simulink model "Q2"  (R2020b)
settings: Solver=VariableStepAuto  StartTime=0.0  StopTime=30  RelTol=1e-3
undefined symbols (not defined in the file): A_num, B_num, C_num, K_fast, K_slow
libraries: simulink x2
settings Model: Creator=asus  LastModifiedBy=asus

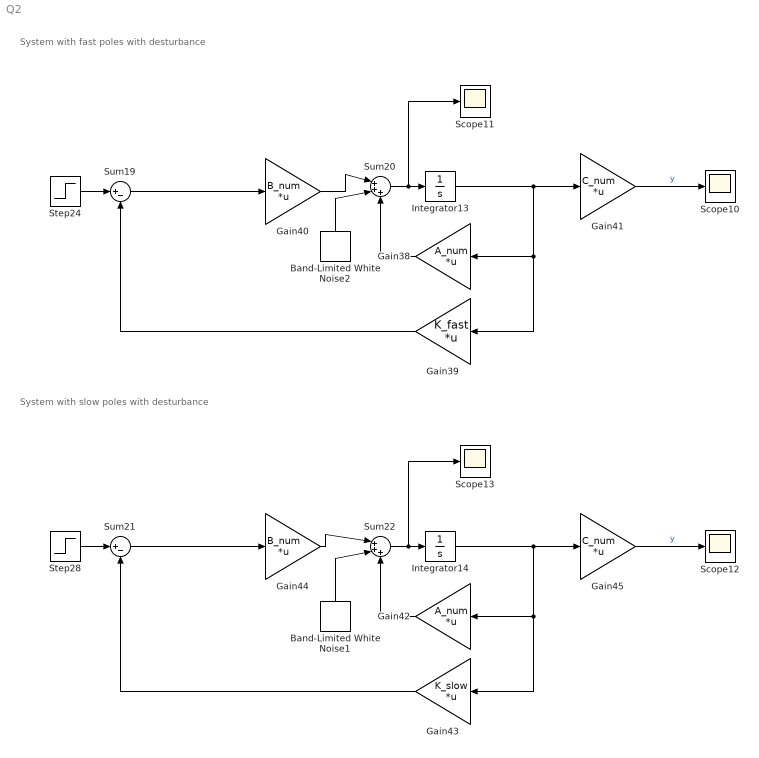
== system Q2 ==
  note: System with fast poles with desturbance
  note: System with slow poles with desturbance
  Band-Limited White Noise1 : simulink/Sources/Band-Limited White Noise  Cov=[0.3; 0.3; 0.3; 0.3]  Ts=10  seed=[456; 456; 456; 456]
  Band-Limited White Noise2 : simulink/Sources/Band-Limited White Noise  Cov=[0.3; 0.3; 0.3; 0.3]  Ts=10  seed=[456; 456; 456; 456]
  Gain38 : Gain  Gain=A_num  Multiplication=Matrix(K*u)
  Gain39 : Gain  Gain=K_fast  Multiplication=Matrix(K*u)
  Gain40 : Gain  Gain=B_num  Multiplication=Matrix(K*u)
  Gain41 : Gain  Gain=C_num  Multiplication=Matrix(K*u)
  Gain42 : Gain  Gain=A_num  Multiplication=Matrix(K*u)
  Gain43 : Gain  Gain=K_slow  Multiplication=Matrix(K*u)
  Gain44 : Gain  Gain=B_num  Multiplication=Matrix(K*u)
  Gain45 : Gain  Gain=C_num  Multiplication=Matrix(K*u)
  Integrator13 : Integrator
  Integrator14 : Integrator
  Scope{10..13} (4 alike) : Scope
  Step24 : Step  SampleTime=0
  Step28 : Step  SampleTime=0
  Sum19 : Sum  Inputs=|+-
  Sum20 : Sum  Inputs=|+++
  Sum21 : Sum  Inputs=|+-
  Sum22 : Sum  Inputs=|+++
  wires:
  Gain43/1 -> Sum21/2
  Gain41/1 -> Scope10/1  "y"
  Gain44/1 -> Sum22/1
  Sum21/1 -> Gain44/1
  Step24/1 -> Sum19/1
  Integrator14/1 -> Gain45/1, Gain43/1, Gain42/1
  Sum20/1 -> Scope11/1, Integrator13/1
  Sum22/1 -> Scope13/1, Integrator14/1
  Step28/1 -> Sum21/1
  Sum19/1 -> Gain40/1
  Gain39/1 -> Sum19/2
  Gain40/1 -> Sum20/1
  Gain45/1 -> Scope12/1  "y"
  Integrator13/1 -> Gain41/1, Gain39/1, Gain38/1
  Gain38/1 -> Sum20/3
  Band-Limited White Noise2/1 -> Sum20/2
  Gain42/1 -> Sum22/3
  Band-Limited White Noise1/1 -> Sum22/2
